simulink model "random_d"  (Simulink 7.1)
settings: Solver=ode45  StartTime=0.0  StopTime=60.0  RelTol=1e-3
settings Model: Creator=Usuario  LastModifiedBy=Usuario  BufferReuse=off
settings OptimizationCC: OptimizeBlockIOStorage=off  BufferReuse=off  ExpressionFolding=off  LocalBlockOutputs=off

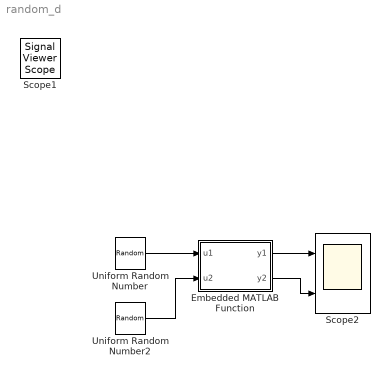
== system random_d ==
  Embedded MATLAB Function : Stateflow chart
  Scope2 : Scope  NumInputPorts=2
      settings: YMin=-5~-5  YMax=5~5  SaveName=ScopeData2
  Uniform Random Number : UniformRandomNumber  Minimum=0  SampleTime=0
  Uniform Random Number2 : UniformRandomNumber  Minimum=0  Seed=1  SampleTime=0
  Scope1 : SignalViewerScope  IOType=viewer  RefreshTime=0.035000
  wires:
  Uniform Random Number/1 -> Embedded MATLAB Function/1(u1)
  Embedded MATLAB Function/1(y1) -> Scope2/1
  Embedded MATLAB Function/2(y2) -> Scope2/2
  Uniform Random Number2/1 -> Embedded MATLAB Function/2(u2)

== matlab function Embedded MATLAB Function ==
  data: u1 input double; y1 output double; u2 input double; y2 output double
function [y1,y2] = sumaresta(u1,u2)
% This block supports the Embedded MATLAB subset.
% See the help menu for details. 

y1 = u1+u2;
y2 = u1-u2;
